simulink model "vcm_plant"  (R2022b)
settings: Solver=ode45  StartTime=0.0  StopTime=0.06  RelTol=1e-3
settings Model: Creator=dohyunseo  LastModifiedBy=dohyunseo

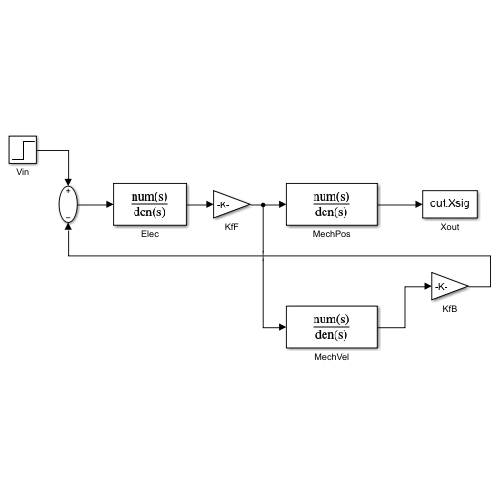
[thumbnail: Simulink's stored preview of the top-level diagram]
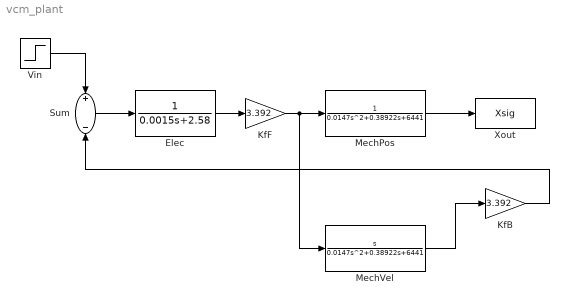
== system vcm_plant ==
  Elec : TransferFcn  Denominator=[0.0015 2.58]
  KfB : Gain  Gain=3.392
  KfF : Gain  Gain=3.392
  MechPos : TransferFcn  Denominator=[0.0147 0.38922 6441]
  MechVel : TransferFcn  Numerator=[1 0]  Denominator=[0.0147 0.38922 6441]
  Sum : Sum  Inputs=+-
  Vin : Step  Time=0  SampleTime=0
  Xout : ToWorkspace  VariableName=Xsig  SaveFormat=Timeseries  SampleTime=-1
  wires:
  Vin/1 -> Sum/1
  Sum/1 -> Elec/1
  Elec/1 -> KfF/1
  KfF/1 -> MechPos/1, MechVel/1
  MechPos/1 -> Xout/1
  MechVel/1 -> KfB/1
  KfB/1 -> Sum/2
